simulink model "test_cs"  (Simulink 8.9)
settings: Solver=ode5  StartTime=0.0  StopTime=290  FixedStep=1/20  RelTol=1e-3
model workspace (MAT data in the model file):
  mbox_table.blocks{1}.src = 'built-in/Subsystem'
  mbox_table.blocks{1}.dest = 'test_cs/Audi_A8_1'
  mbox_table.blocks{1}.mode = 0
  mbox_table.blocks{2}.src = 'simulink/Sinks/Out1'
  mbox_table.blocks{2}.dest = 'test_cs/Audi_A8_1/STATE_Audi_A8_1'
  mbox_table.blocks{2}.mode = 0
  mbox_table.blocks{3}.src = 'PreScanSimulinkLibrary/State'
  mbox_table.blocks{3}.dest = 'test_cs/STATE_Audi_A8_1'
  mbox_table.blocks{3}.mode = 0
  mbox_table.blocks{4}.src = 'PreScanSimulinkLibrary/PathFollower'
  mbox_table.blocks{4}.dest = 'test_cs/Audi_A8_1/PathFollower_1'
  mbox_table.blocks{4}.mode = 0
  mbox_table.blocks{5}.src = 'simulink/Sources/Constant'
  mbox_table.blocks{5}.dest = 'test_cs/Audi_A8_1/pos'
  mbox_table.blocks{5}.mode = 0
  mbox_table.blocks{6}.src = 'PreScanSimulinkLibrary/Trajectories'
  mbox_table.blocks{6}.dest = 'test_cs/Audi_A8_1/Trajectories'
  mbox_table.blocks{6}.mode = 0
  mbox_table.blocks{7}.src = 'simulink/Sources/Constant'
  mbox_table.blocks{7}.dest = 'test_cs/Audi_A8_1/Trajectories/Trajectory_1_Offset'
  mbox_table.blocks{7}.mode = 0
  mbox_table.blocks{8}.src = 'PreScanSimulinkLibrary/Trajectory'
  mbox_table.blocks{8}.dest = 'test_cs/Audi_A8_1/Trajectories/Trajectory_1'
  mbox_table.blocks{8}.mode = 0
  mbox_table.blocks{9}.src = 'PreScanSimulinkLibrary/Traj2State'
  mbox_table.blocks{9}.dest = 'test_cs/Audi_A8_1/Trajectories/Traj2State1'
  mbox_table.blocks{9}.mode = 0
  mbox_table.blocks{10}.src = 'simulink/Sinks/Out1'
  mbox_table.blocks{10}.dest = 'test_cs/Audi_A8_1/Trajectories/State'
  mbox_table.blocks{10}.mode = 0
  mbox_table.blocks{11}.src = 'PreScanSimulinkLibrary/SELF'
  mbox_table.blocks{11}.dest = 'test_cs/SELF_Audi_A8_1'
  mbox_table.blocks{11}.mode = 0
  mbox_table.blocks{12}.src = 'simulink/Sources/In1'
  mbox_table.blocks{12}.dest = 'test_cs/Audi_A8_1/SELF_Audi_A8_1'
  mbox_table.blocks{12}.mode = 0
  mbox_table.blocks{13}.src = 'PreScanSimulinkLibrary/DemuxSELF'
  mbox_table.blocks{13}.dest = 'test_cs/Audi_A8_1/SELF_Demux'
  mbox_table.blocks{13}.mode = 0
  mbox_table.blocks{14}.src = 'PreScanSimulinkLibrary/LaneMarkerSensor'
  mbox_table.blocks{14}.dest = 'test_cs/LaneMarkerSensor_1'
  mbox_table.blocks{14}.mode = 0
  mbox_table.blocks{15}.src = 'simulink/Sources/In1'
  mbox_table.blocks{15}.dest = 'test_cs/Audi_A8_1/LaneMarkerSensor_1'
  mbox_table.blocks{15}.mode = 0
  mbox_table.blocks{16}.src = 'PreScanSimulinkLibrary/LaneMarkerSensor_Data'
  mbox_table.blocks{16}.dest = 'test_cs/Audi_A8_1/LaneMarkerSensor_1_Data'
  mbox_table.blocks{16}.mode = 0
  mbox_table.blocks{17}.src = 'PreScanSimulinkLibrary/CameraSensor_Color_Display'
  mbox_table.blocks{17}.dest = 'test_cs/Audi_A8_1/LaneMarkerSensor_1_Display'
  mbox_table.blocks{17}.mode = 0
  mbox_table.blocks{18}.src = 'PreScanSimulinkLibrary/Simple_Vehicle_Dynamics'
  mbox_table.blocks{18}.dest = 'test_cs/Audi_A8_1/Dynamics_Simple'
  mbox_table.blocks{18}.mode = 0
  mbox_table.blocks{19}.src = 'SimCoreLibrary/SimCoreConfiguration'
  mbox_table.blocks{19}.dest = 'test_cs/SimCoreConfiguration'
  mbox_table.blocks{19}.mode = 0
  mbox_table.blocks{20}.src = 'SimCoreLibrary/Actuators'
  mbox_table.blocks{20}.dest = 'test_cs/Actuators'
  mbox_table.blocks{20}.mode = 0
  mbox_table.blocks{21}.src = 'SimCoreLibrary/SetActuators'
  mbox_table.blocks{21}.dest = 'test_cs/SetActuators'
  mbox_table.blocks{21}.mode = 0
  mbox_table.blocks{22}.src = 'SimCoreLibrary/GetSensors'
  mbox_table.blocks{22}.dest = 'test_cs/GetSensors'
  mbox_table.blocks{22}.mode = 0
  mbox_table.blocks{23}.src = 'SimCoreLibrary/SimCoreInfo'
  mbox_table.blocks{23}.dest = 'test_cs/SimCoreInfo'
  mbox_table.blocks{23}.mode = 0
  mbox_table.blocks{24}.src = 'PreScanSimulinkLibrary/Regenerate'
  mbox_table.blocks{24}.dest = 'test_cs/Regenerate'
  mbox_table.blocks{24}.mode = 0
  mbox_table.blocks{25}.src = 'PreScanSimulinkLibrary/Record for Replay  '
  mbox_table.blocks{25}.dest = 'test_cs/Record for Replay  '
  mbox_table.blocks{25}.mode = 0
  mbox_table.blocks{26}.src = 'PreScanSimulinkLibrary/Open Useful Blocks'
  mbox_table.blocks{26}.dest = 'test_cs/Open Useful Blocks'
  mbox_table.blocks{26}.mode = 0
  mbox_table.blocks{27}.src = 'PreScanSimulinkLibrary/PreScan Options   '
  mbox_table.blocks{27}.dest = 'test_cs/PreScan Options   '
  mbox_table.blocks{27}.mode = 0
  mbox_table.blocks{28}.src = 'built-in/Note'
  mbox_table.blocks{28}.dest = 'test_cs/Version:                  '
  mbox_table.blocks{28}.mode = 0
  mbox_table.blocks{29}.src = 'built-in/Note'
  mbox_table.blocks{29}.dest = 'test_cs/7.0.0'
  mbox_table.blocks{29}.mode = 0
  mbox_table.blocks{30}.src = 'built-in/Note'
  mbox_table.blocks{30}.dest = 'test_cs/Author(s):                '
  mbox_table.blocks{30}.mode = 0
  mbox_table.blocks{31}.src = 'built-in/Note'
  mbox_table.blocks{31}.dest = 'test_cs/N.A.'
  mbox_table.blocks{31}.mode = 0
  mbox_table.blocks{32}.src = 'built-in/Note'
  mbox_table.blocks{32}.dest = 'test_cs/Descriptive text:      '
  mbox_table.blocks{32}.mode = 0
  mbox_table.blocks{33}.src = 'built-in/Note'
  mbox_table.blocks{33}.dest = 'test_cs/N.A.'
  mbox_table.blocks{33}.mode = 0
  mbox_table.blocks{34}.src = 'built-in/Note'
  mbox_table.blocks{34}.dest = 'test_cs/ID
    | 
    | 1'
  mbox_table.blocks{34}.mode = 0
  mbox_table.blocks{35}.src = 'built-in/Note'
  mbox_table.blocks{35}.dest = 'test_cs/OBU-Beacon ID
    | 
    | '
  mbox_table.blocks{35}.mode = 0
  mbox_table.blocks{36}.src = 'built-in/Note'
  mbox_table.blocks{36}.dest = 'test_cs/TypeID
    | 
    | 1'
  mbox_table.blocks{36}.mode = 0
  mbox_table.blocks{37}.src = 'built-in/Note'
  mbox_table.blocks{37}.dest = 'test_cs/TypeTag
    | 
    | Car'
  mbox_table.blocks{37}.mode = 0
  mbox_table.blocks{38}.src = 'built-in/Note'
  mbox_table.blocks{38}.dest = 'test_cs/SD
    | 
    | Y'
  mbox_table.blocks{38}.mode = 0
  mbox_table.blocks{39}.src = 'built-in/Note'
  mbox_table.blocks{39}.dest = 'test_cs/CD
    | 
    | N'
  mbox_table.blocks{39}.mode = 0
  mbox_table.blocks{40}.src = 'built-in/Note'
  mbox_table.blocks{40}.dest = 'test_cs/Name
    | 
    | Audi_A8_1'
  mbox_table.blocks{40}.mode = 0
  mbox_table.blocks{41}.src = 'built-in/Note'
  mbox_table.blocks{41}.dest = 'test_cs/Num ID       OBU-Beacon ID     Type ID      Type Tag             SD        CD             Name                          '
  mbox_table.blocks{41}.mode = 0
  mbox_table.blocks{42}.src = 'built-in/Ground'
  mbox_table.blocks{42}.dest = 'test_cs/Audi_A8_1/Ground_1'
  mbox_table.blocks{42}.mode = 1
  mbox_table.blocks{43}.src = 'built-in/Ground'
  mbox_table.blocks{43}.dest = 'test_cs/Audi_A8_1/Ground_2'
  mbox_table.blocks{43}.mode = 1
  mbox_table.blocks{44}.src = 'built-in/Terminator'
  mbox_table.blocks{44}.dest = 'test_cs/Audi_A8_1/Terminator_1'
  mbox_table.blocks{44}.mode = 1
  mbox_table.blocks{45}.src = 'built-in/Terminator'
  mbox_table.blocks{45}.dest = 'test_cs/Audi_A8_1/Terminator_2'
  mbox_table.blocks{45}.mode = 1
  mbox_table.blocks{46}.src = 'built-in/Ground'
  mbox_table.blocks{46}.dest = 'test_cs/Audi_A8_1/Ground_3'
  mbox_table.blocks{46}.mode = 1
  mbox_table.blocks{47}.src = 'built-in/Terminator'
  mbox_table.blocks{47}.dest = 'test_cs/Audi_A8_1/Terminator_3'
  mbox_table.blocks{47}.mode = 1
  mbox_table.blocks{48}.src = 'built-in/Ground'
  mbox_table.blocks{48}.dest = 'test_cs/Audi_A8_1/Ground_4'
  mbox_table.blocks{48}.mode = 1
  mbox_table.blocks{49}.src = 'built-in/Ground'
  mbox_table.blocks{49}.dest = 'test_cs/Audi_A8_1/Ground_5'
  mbox_table.blocks{49}.mode = 1
  mbox_table.blocks{50}.src = 'built-in/Terminator'
  mbox_table.blocks{50}.dest = 'test_cs/Audi_A8_1/Terminator_4'
  mbox_table.blocks{50}.mode = 1
  mbox_table.blocks{51}.src = 'built-in/Terminator'
  mbox_table.blocks{51}.dest = 'test_cs/Audi_A8_1/Terminator_5'
  mbox_table.blocks{51}.mode = 1
  mbox_table.blocks{52}.src = 'built-in/Terminator'
  mbox_table.blocks{52}.dest = 'test_cs/Audi_A8_1/Terminator_6'
  mbox_table.blocks{52}.mode = 1
  mbox_table.blocks{53}.src = 'built-in/Terminator'
  mbox_table.blocks{53}.dest = 'test_cs/Audi_A8_1/Terminator_7'
  mbox_table.blocks{53}.mode = 1
  mbox_table.blocks{54}.src = 'built-in/Terminator'
  mbox_table.blocks{54}.dest = 'test_cs/Audi_A8_1/Terminator_8'
  mbox_table.blocks{54}.mode = 1
  mbox_table.blocks{55}.src = 'built-in/Terminator'
  mbox_table.blocks{55}.dest = 'test_cs/Audi_A8_1/Terminator_9'
  mbox_table.blocks{55}.mode = 1
  mbox_table.blocks{56}.src = 'built-in/Terminator'
  mbox_table.blocks{56}.dest = 'test_cs/Audi_A8_1/Terminator_10'
  mbox_table.blocks{56}.mode = 1
  mbox_table.blocks{57}.src = 'built-in/Terminator'
  mbox_table.blocks{57}.dest = 'test_cs/Audi_A8_1/Terminator_11'
  mbox_table.blocks{57}.mode = 1
  mbox_table.blocks{58}.src = 'built-in/Terminator'
  mbox_table.blocks{58}.dest = 'test_cs/Audi_A8_1/Terminator_12'
  mbox_table.blocks{58}.mode = 1
  mbox_table.blocks{59}.src = 'built-in/Terminator'
  mbox_table.blocks{59}.dest = 'test_cs/Audi_A8_1/Terminator_13'
  mbox_table.blocks{59}.mode = 1
  mbox_table.blocks{60}.src = 'built-in/Terminator'
  mbox_table.blocks{60}.dest = 'test_cs/Audi_A8_1/Terminator_14'
  mbox_table.blocks{60}.mode = 1
  mbox_table.block_index : java.util.Hashtable (value not decoded)
  mbox_table.lines{1}.sys = 'test_cs'
  mbox_table.lines{1}.line_id = 'L1'
  mbox_table.lines{1}.iport = 'STATE_Audi_A8_1/1'
  mbox_table.lines{1}.oport = 'Audi_A8_1/1'
  mbox_table.lines{1}.mode = 0
  mbox_table.lines{2}.sys = 'test_cs/Audi_A8_1'
  mbox_table.lines{2}.line_id = 'L2'
  mbox_table.lines{2}.iport = 'PathFollower_1/1'
  mbox_table.lines{2}.oport = 'pos/1'
  mbox_table.lines{2}.mode = 0
  mbox_table.lines{3}.sys = 'test_cs/Audi_A8_1/Trajectories'
  mbox_table.lines{3}.line_id = 'L3'
  mbox_table.lines{3}.iport = 'Traj2State1/1'
  mbox_table.lines{3}.oport = 'Trajectory_1/1'
  mbox_table.lines{3}.mode = 0
  mbox_table.lines{4}.sys = 'test_cs/Audi_A8_1/Trajectories'
  mbox_table.lines{4}.line_id = 'L4'
  mbox_table.lines{4}.iport = 'Traj2State1/2'
  mbox_table.lines{4}.oport = 'Trajectory_1_Offset/1'
  mbox_table.lines{4}.mode = 0
  mbox_table.lines{5}.sys = 'test_cs/Audi_A8_1/Trajectories'
  mbox_table.lines{5}.line_id = 'L5'
  mbox_table.lines{5}.iport = 'State/1'
  mbox_table.lines{5}.oport = 'Traj2State1/1'
  mbox_table.lines{5}.mode = 0
  mbox_table.lines{6}.sys = 'test_cs'
  mbox_table.lines{6}.line_id = 'L6'
  mbox_table.lines{6}.iport = 'Audi_A8_1/1'
  mbox_table.lines{6}.oport = 'SELF_Audi_A8_1/1'
  mbox_table.lines{6}.mode = 0
  mbox_table.lines{7}.sys = 'test_cs/Audi_A8_1'
  mbox_table.lines{7}.line_id = 'L7'
  mbox_table.lines{7}.iport = 'SELF_Demux/1'
  mbox_table.lines{7}.oport = 'SELF_Audi_A8_1/1'
  mbox_table.lines{7}.mode = 0
  mbox_table.lines{8}.sys = 'test_cs/Audi_A8_1'
  mbox_table.lines{8}.line_id = 'L8'
  mbox_table.lines{8}.iport = 'LaneMarkerSensor_1_Display/1'
  mbox_table.lines{8}.oport = 'LaneMarkerSensor_1_Data/2'
  mbox_table.lines{8}.mode = 0
  mbox_table.lines{9}.sys = 'test_cs/Audi_A8_1'
  mbox_table.lines{9}.line_id = 'L9'
  mbox_table.lines{9}.iport = 'LaneMarkerSensor_1_Display/2'
  mbox_table.lines{9}.oport = 'LaneMarkerSensor_1_Data/3'
  mbox_table.lines{9}.mode = 0
  mbox_table.lines{10}.sys = 'test_cs/Audi_A8_1'
  mbox_table.lines{10}.line_id = 'L10'
  mbox_table.lines{10}.iport = 'LaneMarkerSensor_1_Display/3'
  mbox_table.lines{10}.oport = 'LaneMarkerSensor_1_Data/4'
  mbox_table.lines{10}.mode = 0
  mbox_table.lines{11}.sys = 'test_cs/Audi_A8_1'
  mbox_table.lines{11}.line_id = 'L11'
  mbox_table.lines{11}.iport = 'LaneMarkerSensor_1_Data/1'
  mbox_table.lines{11}.oport = 'LaneMarkerSensor_1/1'
  mbox_table.lines{11}.mode = 0
  mbox_table.lines{12}.sys = 'test_cs'
  mbox_table.lines{12}.line_id = 'L12'
  mbox_table.lines{12}.iport = 'Audi_A8_1/2'
  mbox_table.lines{12}.oport = 'LaneMarkerSensor_1/1'
  mbox_table.lines{12}.mode = 0
  mbox_table.lines{13}.sys = 'test_cs/Audi_A8_1'
  mbox_table.lines{13}.line_id = 'l9'
  mbox_table.lines{13}.iport = 'Dynamics_Simple/1'
  mbox_table.lines{13}.oport = 'PathFollower_1/1'
  mbox_table.lines{13}.mode = 0
  mbox_table.lines{14}.sys = 'test_cs/Audi_A8_1'
  mbox_table.lines{14}.line_id = 'L14'
  mbox_table.lines{14}.iport = 'Dynamics_Simple/2'
  mbox_table.lines{14}.oport = 'PathFollower_1/2'
  mbox_table.lines{14}.mode = 0
  mbox_table.lines{15}.sys = 'test_cs/Audi_A8_1'
  mbox_table.lines{15}.line_id = 'L15'
  mbox_table.lines{15}.iport = 'Dynamics_Simple/3'
  mbox_table.lines{15}.oport = 'PathFollower_1/3'
  mbox_table.lines{15}.mode = 0
  mbox_table.lines{16}.sys = 'test_cs/Audi_A8_1'
  mbox_table.lines{16}.line_id = 'L16'
  mbox_table.lines{16}.iport = 'Dynamics_Simple/4'
  mbox_table.lines{16}.oport = 'PathFollower_1/4'
  mbox_table.lines{16}.mode = 0
  mbox_table.lines{17}.sys = 'test_cs/Audi_A8_1'
  mbox_table.lines{17}.line_id = 'L17'
  mbox_table.lines{17}.iport = 'Dynamics_Simple/6'
  mbox_table.lines{17}.oport = 'PathFollower_1/5'
  mbox_table.lines{17}.mode = 0
  mbox_table.lines{18}.sys = 'test_cs/Audi_A8_1'
  mbox_table.lines{18}.line_id = 'L18'
  mbox_table.lines{18}.iport = 'STATE_Audi_A8_1/1'
  mbox_table.lines{18}.oport = 'Dynamics_Simple/1'
  mbox_table.lines{18}.mode = 0
  mbox_table.lines{19}.sys = 'test_cs/Audi_A8_1'
  mbox_table.lines{19}.line_id = 'l1'
  mbox_table.lines{19}.iport = 'Dynamics_Simple/5'
  mbox_table.lines{19}.oport = 'Ground_1/1'
  mbox_table.lines{19}.mode = 1
  mbox_table.lines{20}.sys = 'test_cs/Audi_A8_1'
  mbox_table.lines{20}.line_id = 'l2'
  mbox_table.lines{20}.iport = 'Dynamics_Simple/7'
  mbox_table.lines{20}.oport = 'Ground_2/1'
  mbox_table.lines{20}.mode = 1
  mbox_table.lines{21}.sys = 'test_cs/Audi_A8_1'
  mbox_table.lines{21}.line_id = 'l3'
  mbox_table.lines{21}.iport = 'Terminator_1/1'
  mbox_table.lines{21}.oport = 'Dynamics_Simple/2'
  mbox_table.lines{21}.mode = 1
  mbox_table.lines{22}.sys = 'test_cs/Audi_A8_1'
  mbox_table.lines{22}.line_id = 'l4'
  mbox_table.lines{22}.iport = 'Terminator_2/1'
  mbox_table.lines{22}.oport = 'Dynamics_Simple/3'
  mbox_table.lines{22}.mode = 1
  mbox_table.lines{23}.sys = 'test_cs/Audi_A8_1'
  mbox_table.lines{23}.line_id = 'l5'
  mbox_table.lines{23}.iport = 'Gain4/1'
  mbox_table.lines{23}.oport = 'Ground_3/1'
  mbox_table.lines{23}.mode = 1
  mbox_table.lines{24}.sys = 'test_cs/Audi_A8_1'
  mbox_table.lines{24}.line_id = 'l6'
  mbox_table.lines{24}.iport = 'Terminator_3/1'
  mbox_table.lines{24}.oport = 'Gain4/1'
  mbox_table.lines{24}.mode = 1
  mbox_table.lines{25}.sys = 'test_cs/Audi_A8_1'
  mbox_table.lines{25}.line_id = 'l7'
  mbox_table.lines{25}.iport = 'PathFollower_1/2'
  mbox_table.lines{25}.oport = 'Ground_4/1'
  mbox_table.lines{25}.mode = 1
  mbox_table.lines{26}.sys = 'test_cs/Audi_A8_1'
  mbox_table.lines{26}.line_id = 'l8'
  mbox_table.lines{26}.iport = 'PathFollower_1/4'
  mbox_table.lines{26}.oport = 'Ground_5/1'
  mbox_table.lines{26}.mode = 1
  mbox_table.lines{27}.sys = 'test_cs/Audi_A8_1'
  mbox_table.lines{27}.line_id = 'l9'
  mbox_table.lines{27}.iport = 'Terminator_4/1'
  mbox_table.lines{27}.oport = 'PathFollower_1/1'
  mbox_table.lines{27}.mode = 1
  mbox_table.lines{28}.sys = 'test_cs/Audi_A8_1'
  mbox_table.lines{28}.line_id = 'l10'
  mbox_table.lines{28}.iport = 'Terminator_5/1'
  mbox_table.lines{28}.oport = 'PathFollower_1/6'
  mbox_table.lines{28}.mode = 1
  mbox_table.lines{29}.sys = 'test_cs/Audi_A8_1'
  mbox_table.lines{29}.line_id = 'l11'
  mbox_table.lines{29}.iport = 'Terminator_6/1'
  mbox_table.lines{29}.oport = 'PathFollower_1/7'
  mbox_table.lines{29}.mode = 1
  mbox_table.lines{30}.sys = 'test_cs/Audi_A8_1'
  mbox_table.lines{30}.line_id = 'l12'
  mbox_table.lines{30}.iport = 'Terminator_7/1'
  mbox_table.lines{30}.oport = 'SELF_Demux/3'
  mbox_table.lines{30}.mode = 1
  mbox_table.lines{31}.sys = 'test_cs/Audi_A8_1'
  mbox_table.lines{31}.line_id = 'l13'
  mbox_table.lines{31}.iport = 'Terminator_8/1'
  mbox_table.lines{31}.oport = 'SELF_Demux/4'
  mbox_table.lines{31}.mode = 1
  mbox_table.lines{32}.sys = 'test_cs/Audi_A8_1'
  mbox_table.lines{32}.line_id = 'l14'
  mbox_table.lines{32}.iport = 'Terminator_9/1'
  mbox_table.lines{32}.oport = 'SELF_Demux/5'
  mbox_table.lines{32}.mode = 1
  mbox_table.lines{33}.sys = 'test_cs/Audi_A8_1'
  mbox_table.lines{33}.line_id = 'l15'
  mbox_table.lines{33}.iport = 'Terminator_10/1'
  mbox_table.lines{33}.oport = 'SELF_Demux/7'
  mbox_table.lines{33}.mode = 1
  mbox_table.lines{34}.sys = 'test_cs/Audi_A8_1'
  mbox_table.lines{34}.line_id = 'l16'
  mbox_table.lines{34}.iport = 'Terminator_11/1'
  mbox_table.lines{34}.oport = 'SELF_Demux/8'
  mbox_table.lines{34}.mode = 1
  mbox_table.lines{35}.sys = 'test_cs/Audi_A8_1'
  mbox_table.lines{35}.line_id = 'l17'
  mbox_table.lines{35}.iport = 'Terminator_12/1'
  mbox_table.lines{35}.oport = 'SELF_Demux/9'
  mbox_table.lines{35}.mode = 1
  mbox_table.lines{36}.sys = 'test_cs/Audi_A8_1'
  mbox_table.lines{36}.line_id = 'l18'
  mbox_table.lines{36}.iport = 'Terminator_13/1'
  mbox_table.lines{36}.oport = 'SELF_Demux/11'
  mbox_table.lines{36}.mode = 1
  mbox_table.lines{37}.sys = 'test_cs/Audi_A8_1'
  mbox_table.lines{37}.line_id = 'l19'
  mbox_table.lines{37}.iport = 'Terminator_14/1'
  mbox_table.lines{37}.oport = 'Trajectories/1'
  mbox_table.lines{37}.mode = 1
  mbox_table.line_index : java.util.Hashtable (value not decoded)
  mbox_table.next_linenr = 19
  mbox_table.next_termlinenr = 20
  model_closed = 0
  sim_status = 0
PreLoadFcn:
  | check_NUTS_defined;
  | 
  | assignin('base',['model_closed_' bdroot],false);
InitFcn:
  | PreScanExperimentInitFcn(bdroot)
StopFcn:
  | PreScanExperimentStopFcn(bdroot)
values from neighbouring files (symbols this model uses):
  a11 = -2*(cf*Lf^2+cr*Lr^2)/(Iz*Vx)    (= -13.1812002432)    [lkas.m]
  a12 = 2*(cf*Lf-cr*Lr)/Iz    (= -69.3863961559)    [lkas.m]
  a13 = -2*(cf*Lf-cr*Lr)/(Iz*Vx)    (= 3.56925906152)    [lkas.m]
  a16 = 2*cf*Lf/Iz    (= 45.3838814736)    [lkas.m]
  a31 = 2*(-cf*Lf+cr*Lr)/(M*Vx)    (= 7.3463980464)    [lkas.m]
  a32 = 2*(cf+cr)/M    (= 213.298901099)    [lkas.m]
  a33 = -2*(cf+cr)/(M*Vx)    (= -10.9721656944)    [lkas.m]
  a36 = 2*cf/M    (= 79.8384615385)    [lkas.m]
  K = acker(A, B, [-10+10i -10-10i -10 -10])    [lkas.m]
  L = L'    [lkas.m]
undefined symbols (not defined in the file or in its folder): InitImageOutputDir
libraries: simulink x18, PreScanSimulinkLibrary x6, simulink_extras x3
(part 1 of 3)
CloseFcn:
  | evalin('base',['clear model_closed_' bdroot]);
settings Model: Creator=PRESCAN  LastModifiedBy=edward
settings OptimizationCC: ExpressionDepthLimit=2147483647  InitFltsAndDblsToZero=on
settings DebuggingCC: SaveWithParameterizedLinksMsg=none  SignalResolutionControl=TryResolveAllWithWarning  MultiTaskDSMMsg=warning  MultiTaskCondExecSysMsg=none
settings GRTTargetCC: TargetFcnLib=ansi_tfl_tmw.mat

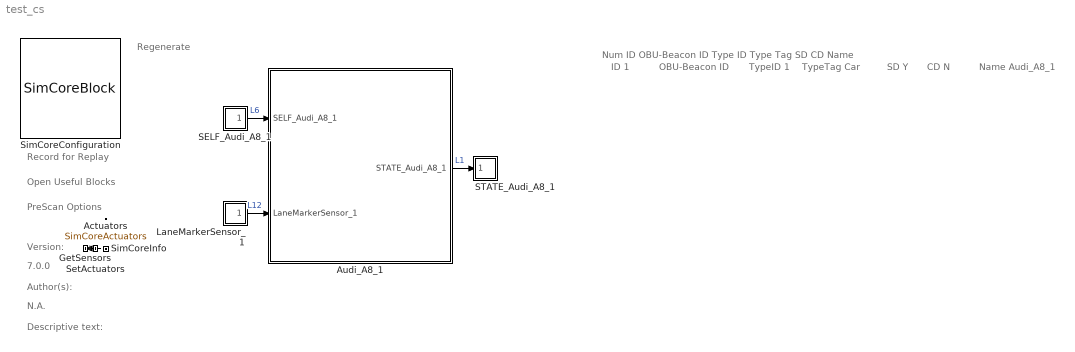
== system test_cs ==
  note: Regenerate
  note: Record for Replay
  note: Open Useful Blocks
  note: PreScan Options
  note: Version:
  note: 7.0.0
  note: Author(s):
  note: N.A.
  note: Descriptive text:
  note: ID
      |
      | 1
  note: OBU-Beacon ID
  note: TypeID
      |
      | 1
  note: TypeTag
      |
      | Car
  note: SD
      |
      | Y
  note: CD
      |
      | N
  note: Name
      |
      | Audi_A8_1
  note: Num ID OBU-Beacon ID Type ID Type Tag SD CD Name
  Actuators : DataStoreMemory  DataStoreName=SimCoreActuators  InitialValue=zeros(15,1)  ShowAdditionalParam=off
  Audi_A8_1 : Subsystem  Tag=WorldObjectSubSystem  InitFcn=UniqueId = '13';
      mask Display: image(imread('Audi_A8.jpg'));color('white');text(0,0,' ID=1\n')
  GetSensors : Subsystem  Tag=GetSensors  mask(PreScan Simulation Core Block){NrOfSensors=8, TimeStep=1/20}
      mask prompts: NrOfSensors "Number of sensor values"; TimeStep "Timestep [s]"
      mask help:
      | Please do not remove this block from the PreScan compilation sheet,
      | as it contains essential configuration parameters for a PreScan simulation.
      settings: DeleteFcn=PreScanBlockDeleteFcn;
  LaneMarkerSensor_1 : Subsystem  Tag=LaneMarkerSensor  mask(PreScan Source Block: Lane Marker Sensor){}
      mask help: The Lane Marker Sensor provides information relating the sensor to the lane markers on the road.
      settings: DeleteFcn=PreScanBlockDeleteFcn;
      mask Help: eval('openHelp(457)')
      mask Display: image(imread('LaneMarkerSensorSL.png'))
  SELF_Audi_A8_1 : Subsystem  Tag=SELF  mask(PreScan Source Block: SELF){PortName=SELF_Audi_A8_1, PortIndex=0, PortWidth=8, TimeStep=1/20}
      mask prompts: PortName "Auto-Assigned: Port Name [-]"; PortIndex "Auto-Assigned: Port Index [-]"; PortWidth "Auto-Assigned: Port Dimensions"; TimeStep "Auto-Assigned: Upload Period [s]"
      mask help:
      | The SELF port shows (state) information of the actor itself. The outputs are position in the experiment's axis system and the GPS coordinates, and the object's absolute velocity and compass heading.
      |
      | For more information, please click Help.
      settings: DeleteFcn=PreScanBlockDeleteFcn;
      mask Help: eval('openHelp(462)')
      mask Display: image(imread('GPS.png'))
  STATE_Audi_A8_1 : Subsystem  Tag=State  mask(PreScan Sink Block: State){x0=-466.9761730372511, y0=-32.058094010780337, z0=0.55, Roll0=0, Pitch0=0, Yaw0=0, TimeStep=1/20}
      mask prompts: x0 "Ini x-position VEHICLE wrt GLOBAL axis system [m]"; y0 "Ini y-position VEHICLE wrt GLOBAL axis system [m]"; z0 "Ini z-position VEHICLE wrt GLOBAL axis system [m]"; Roll0 "Ini roll-angle BODY wrt VEHICLE axis system [deg]"; Pitch0 "Ini pitch-angle BODY wrt VEHICLE axis system [deg]"; Yaw0 "Ini yaw-angle VEHICLE wrt GLOBAL axis system [deg]"; TimeStep "Time Step [s]"
      mask help:
      | The Actor State contains a vector signal of size (9x1), containing the following signals:
      |
      | -  Position                  (x,y,z)                                     [m]
      | -  Velocity                  (vx,vy,vz)                               [m/s]
      | -  Angles                    (Roll, Pitch, Yaw)                   [rad]
      |
      | The Actor state is defined in the global axis system.
      | The state is superponed on the Initial position defined in the GUI.
      |
      | For more information, please click Help.
      settings: DeleteFcn=PreScanBlockDeleteFcn;
      mask Help: eval('openHelp(222)')
      mask Display: image(imread('State.png'))
  SetActuators : Subsystem  Tag=SetActuators  mask(PreScan Simulation Core Block){TimeStep=1/20, NrOfActuators=15}
      mask prompts: TimeStep "Timestep [s]"; NrOfActuators "Number of actuator values"
      mask help:
      | Please do not remove this block from the PreScan compilation sheet,
      | as it contains essential configuration parameters for a PreScan simulation.
      settings: DeleteFcn=PreScanBlockDeleteFcn;
  SimCoreConfiguration : M-S-Function  Tag=SimCoreConfiguration  Description=FE4822352E09E935CCF95F68F07A56B5C1887AE4C351415F02894CADC90007F4  FunctionName=SimCoreBlock  Parameters=ExperimentXML PortsXML SimulationCore HostName CheckStart EnableLog RfR EnableGPUAccel ShowComputationTime  mask(PreScan Simulation Core Configurator){SimulationCore=NUTS, HostName=0, CheckStart=0, prescanversion='7.0.0', EnableLog=off, RfR=0, EnableGPUAccel=off, ShowComputationTime=off}
      mask prompts: SimulationCore "Simulation Core"; HostName "Simulation Host"; CheckStart "Show START Dialog"; prescanversion "PreScan Version"; EnableLog "Create TA Log"; RfR "Record for Replay"; EnableGPUAccel "Enable GPU Acceleration"; ShowComputationTime "Show ComputationTime Scope"
      mask help:
      | Please do not remove this block from the PreScan compilation sheet,
      | as it contains essential configuration parameter for a PreScan simulation.
      mask init:
      | model = bdroot;
      | ExperimentXML = [model(1:end-3) '.pex'];
      | PortsXML = [model '_ports.pcd'];
      settings: DeleteFcn=PreScanBlockDeleteFcn;  ModelCloseFcn=assignin('base',['model_closed_' bdroot],true);
      mask Help: eval('openHelp(812)')
      mask Display: image(imread('prescanlogo.ico'))
  SimCoreInfo : Subsystem  Tag=SimCoreInfo
  wires:
  SetActuators/1(dummy) -> GetSensors/1(dummy)
  Audi_A8_1/1(STATE_Audi_A8_1) -> STATE_Audi_A8_1/1(State)  "L1"
  SELF_Audi_A8_1/1(U) -> Audi_A8_1/1(SELF_Audi_A8_1)  "L6"
  LaneMarkerSensor_1/1(U) -> Audi_A8_1/2(LaneMarkerSensor_1)  "L12"

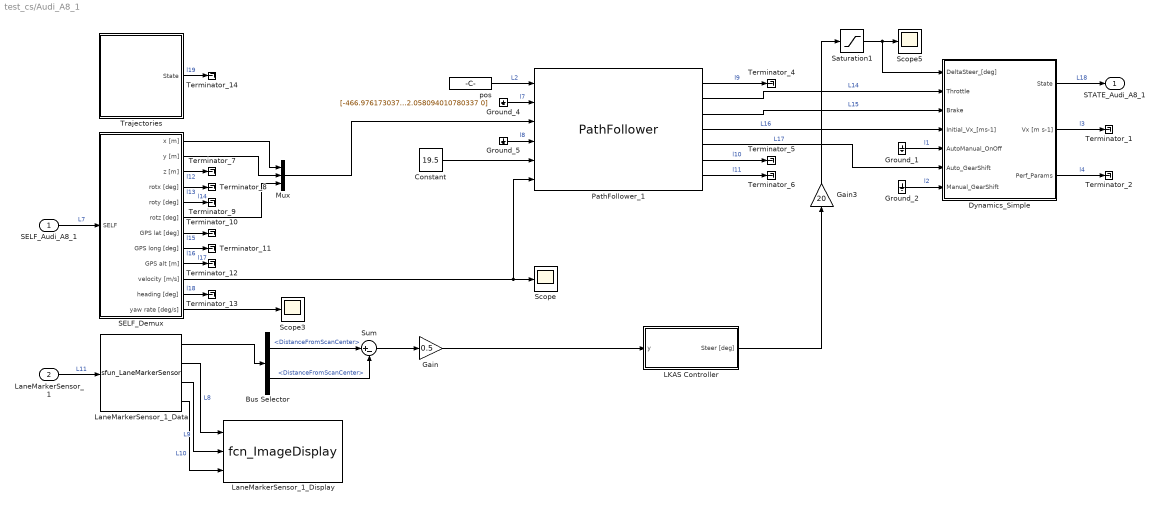
== system test_cs/Audi_A8_1 ==
  SELF_Audi_A8_1 : Inport  Tag=SELFInport
  LaneMarkerSensor_1 : Inport  Tag=LaneMarkerSensorInport  Port=2  SampleTime=1/20
  Bus Selector : BusSelector  OutputSignals=ScanAtDistance1.LeftCurbIntersection.DistanceFromScanCenter,ScanAtDistance1.RightCurbIntersection.DistanceFromScanCenter
  Constant : Constant  Value=19.5
  Dynamics_Simple : Subsystem  Tag=Simple_Vehicle_Dynamics  mask(PreScan Block: Simple Dynamics){TimeStep=1/20, ComputationMode=Continuous_Time}
      mask prompts: TimeStep "Auto assigned: Time Step [s]"; ComputationMode "Computation mode:"
      mask help:
      | The Simple Dynamics Model is selected in the GUI to simulate vehicle dynamics behavior.
      |
      | The Simple Dynamics Model is completely open to the user. The parameters of this model can be set in the Simple Dynamics dialog in the GUI.
      |
      | For more information, please click Help.
      mask init:
      | p = SimpleDyn_pars;
      settings: DeleteFcn=PreScanBlockDeleteFcn;
      mask Help: eval('openHelp(220)')
      mask Display:
      | image(imread('SimpleDyn.png'))
      | port_label('input', 1, '{\delta}_S_t_ _e_e_r [deg]','texmode','on')
      | port_label('input', 2, 'Throttle [%]')
      | port_label('input', 3, 'Brake Pres [bar]')
      | port_label('input', 4, 'V_0 [ms-1]','texmode','on')
      | port_label('input', 5, 'Auto=[0]/Manual=[1]')
      | port_label('input', 6, 'Auto_GearShift')
      | port_label('input', 7, 'Manual_GearShift')
      | port_label('output', 1, 'State')
      | port_label('output', 2, 'Vx [ms-1]')
      | port_label('output', 3, 'Perf Params')
  Gain : Gain  Gain=0.5
  Gain3 : Gain  Gain=20
  Ground_{1..2,4..5} (4 alike) : Ground
  LKAS Controller : Subsystem
  LaneMarkerSensor_1_Data : S-Function  Tag=LaneMarkerSensor_Data  LoadFcn=load('LaneMarkerSensorBusses.mat');  FunctionName=sfun_LaneMarkerSensor  Parameters=[VerticalResolution HorizontalResolution] FrameRate SensorName OutputReferenceImage SharedMemTag SharedMemDataTag  SFunctionDeploymentMode=off  EnableBusSupport=on  mask{HorizontalResolution=320, VerticalResolution=240, FrameRate=20, SensorName=LaneMarkerSensor_1, OutputReferenceImage=on, SharedMemTag=LaneMarkerSensor_1_monoBeam_viewer_RGB, SharedMemDataTag=LaneMarkerSensor_1_monoBeam_viewer_LMS_Data}
      mask prompts: HorizontalResolution "User Specified: Horizontal Resolution [pixels]"; VerticalResolution "User Specified: Vertical Resolution [pixels]"; FrameRate "User Specified: Frame Rate [Hz]"; SensorName "User Specified: Lane Marker Sensor Name"; OutputReferenceImage "User Specified: Output Reference Image"; SharedMemTag "Tag for shared memory for lane marker img"; SharedMemDataTag "Tag for shared memory data"
      mask init:
      | DataPort = 1;
      | if OutputReferenceImage==1
      |     Rport = 2;
      |     Gport = 3;
      |     Bport = 4;
      |     RportName = 'Ref. Image R';
      |     GportName = 'Ref. Image G';
      |     BportName = 'Ref. Image B';
      | else
      |     Rport = 1;
      |     Gport = 1;
      |     Bport = 1;
      |     RportName = '';
      |     GportName = '';
      |     BportName = '';
      | end
      settings: DeleteFcn=PreScanBlockDeleteFcn;
      mask Display:
      | port_label('output',DataPort,'Detection Data')
      | port_label('output',Rport,RportName)
      | port_label('output',Gport,GportName)
      | port_label('output',Bport,BportName)
  LaneMarkerSensor_1_Display : M-S-Function  Tag=CameraSensor_Color_Display  InitFcn=InitImageOutputDir(gcb);  FunctionName=fcn_ImageDisplay  Parameters=SensorName EnableDisplay EnablePosition DisplayPosition FigureHandle SaveResults BitmapFormat TempOutputDir CameraType  mask(PreScan Color Display Block){SensorName=LaneMarkerSensor_1, EnableDisplay=on, EnablePosition=off, DisplayPosition=[10 10 320 240], FigureHandle=100, SaveResults=off, Format=PNG, TempOutputDir=0, CameraType=Mono}
      mask prompts: SensorName "User Specified: Title of Display"; EnableDisplay "Active"; EnablePosition "Set Display window position"; DisplayPosition "Display window position [xpos ypos width height]"; FigureHandle "Unique Handle"; SaveResults "Save results"; TempOutputDir "OutputDir"; CameraType "Camera Type"
      mask help: This block displays the RGB output of a PreScan camera sensor.
      mask init:
      | if EnableDisplay
      |     EnableString='';
      |     EnableColor='gray';
      | else
      |     EnableString='INACTIVE';
      |     EnableColor='red';
      | end
      | switch Format
      |     case 1
      |         BitmapFormat = 'png';
      |     case 2
      |         BitmapFormat = 'bmp';
      |     case 3
      |         BitmapFormat = 'jpg';
      | end 
      | if CameraType==1
      |     CameraTypeName='MONO';
      |     PortNumber=0;
      | else
      |     CameraTypeName='STEREO';
      |     PortNumber=3;
      | end
      settings: DeleteFcn=PreScanBlockDeleteFcn;  ModelCloseFcn=fcn_ImageDisplay_ModelCloseFcn
      mask Help: eval('openHelp(457)')
      mask Callback EnablePosition:
      | MV=get_param(gcb,'MaskVisibilities');
      | if strcmp(get_param(gcb,'EnablePosition'),'on')
      |     MV{4}='on';
      | else
      |     MV{4}='off';
      | end
      | set_param(gcb,'MaskVisibilities',MV);
      mask TypeOptions Format: PNG | BMP | JPG
      mask TypeOptions CameraType: Mono | Stereo
      mask Display:
      | color(EnableColor);
      | fprintf('%s\n DISPLAY:\n Color \n %s',EnableString,SensorName)
      | port_label('input',1,'R')
      | port_label('input',2,'G')
      | port_label('input',3,'B')
      | port_label('input',PortNumber+1,'R')
      | port_label('input',PortNumber+2,'G')
      | port_label('input',PortNumber+3,'B')
  Mux : Mux  Inputs=3
  PathFollower_1 : PreScanSimulinkLibrary/PathFollower  Tag=pathFollower  FileName='Trajectory_1.mat'  TunableSteeringGain=1  XShifting_wrt_COG=0
  SELF_Demux : Subsystem  Tag=DemuxSELF  mask(PreScan Demux Block:){}
      settings: DeleteFcn=PreScanBlockDeleteFcn;
      mask Display:
      | port_label('output',1,'x [m]')
      | port_label('output',2,'y [m]')
      | port_label('output',3,'z [m]','texmode','on')
      | port_label('output',4,'Rotx [deg]','texmode','on')
      | port_label('output',5,'Roty [deg]','texmode','on')
      | port_label('output',6,'Rotz [deg]','texmode','on')
      | port_label('output',7,'GPS lat [deg]','texmode','on')
      | port_label('output',8,'GPS long [deg]','texmode','on')
      | port_label('output',9,'GPS alt [m]','texmode','on')
      | port_label('output',10,'Velocity [m/s]')
      | port_label('output',11,'Heading [deg]')
      | port_label('output',12,'Yaw rate [deg/s]')
  Saturation1 : Saturate  UpperLimit=400  LowerLimit=-400
  Scope : Scope
  Scope3 : Scope
  Scope5 : Scope
  Sum : Sum  Inputs=|+-
  Terminator_{1..2,4..14} (13 alike) : Terminator
  Trajectories : Subsystem  Tag=Trajectories  mask(PreScan Source Block: Trajectories){}
      mask help:
      | The Trajectory block contains the trajectories defined in the PreScan Experiment Editor. The output of the trajectory block is the (vehicle) State.
      |
      | For more information, please click Help.
      settings: DeleteFcn=PreScanBlockDeleteFcn;
      mask Help: eval('openHelp(312)')
      mask Display: image(imread('Trajectory.png'));
  pos : Constant  Tag=pos  Value=[-466.9761730372511 -32.058094010780337 0]
  STATE_Audi_A8_1 : Outport  Tag=StateOutport
  wires:
  LaneMarkerSensor_1_Data/1 -> Bus Selector/1
  Mux/1 -> PathFollower_1/3
  SELF_Demux/1(x [m]) -> Mux/1
  SELF_Demux/2(y [m]) -> Mux/2
  SELF_Demux/6(rotz [deg]) -> Mux/3
  SELF_Demux/10(velocity [m/s]) -> PathFollower_1/6, Scope/1
  Bus Selector/1 -> Sum/1  "<DistanceFromScanCenter>"
  Bus Selector/2 -> Sum/2  "<DistanceFromScanCenter>"
  Sum/1 -> Gain/1
  Constant/1 -> PathFollower_1/5
  Gain3/1 -> Saturation1/1
  Saturation1/1 -> Scope5/1, Dynamics_Simple/1(DeltaSteer_[deg])
  SELF_Demux/12(yaw rate [deg/s]) -> Scope3/1
  pos/1 -> PathFollower_1/1  "L2"
  SELF_Audi_A8_1/1 -> SELF_Demux/1(SELF)  "L7"
  LaneMarkerSensor_1_Data/2 -> LaneMarkerSensor_1_Display/1  "L8"
  LaneMarkerSensor_1_Data/3 -> LaneMarkerSensor_1_Display/2  "L9"
  LaneMarkerSensor_1_Data/4 -> LaneMarkerSensor_1_Display/3  "L10"
  LaneMarkerSensor_1/1 -> LaneMarkerSensor_1_Data/1  "L11"
  PathFollower_1/2 -> Dynamics_Simple/2(Throttle)  "L14"
  PathFollower_1/3 -> Dynamics_Simple/3(Brake)  "L15"
  PathFollower_1/4 -> Dynamics_Simple/4(Initial_Vx_[ms-1])  "L16"
  PathFollower_1/5 -> Dynamics_Simple/6(Auto_GearShift)  "L17"
  Dynamics_Simple/1(State) -> STATE_Audi_A8_1/1  "L18"
  Ground_1/1 -> Dynamics_Simple/5(AutoManual_OnOff)  "l1"
  Ground_2/1 -> Dynamics_Simple/7(Manual_GearShift)  "l2"
  Dynamics_Simple/2(Vx [m s-1]) -> Terminator_1/1  "l3"
  Dynamics_Simple/3(Perf_Params) -> Terminator_2/1  "l4"
  Ground_4/1 -> PathFollower_1/2  "l7"
  Ground_5/1 -> PathFollower_1/4  "l8"
  PathFollower_1/1 -> Terminator_4/1  "l9"
  PathFollower_1/6 -> Terminator_5/1  "l10"
  PathFollower_1/7 -> Terminator_6/1  "l11"
  SELF_Demux/3(z [m]) -> Terminator_7/1  "l12"
  SELF_Demux/4(rotx [deg]) -> Terminator_8/1  "l13"
  SELF_Demux/5(roty [deg]) -> Terminator_9/1  "l14"
  SELF_Demux/7(GPS lat [deg]) -> Terminator_10/1  "l15"
  SELF_Demux/8(GPS long [deg]) -> Terminator_11/1  "l16"
  SELF_Demux/9(GPS alt [m]) -> Terminator_12/1  "l17"
  SELF_Demux/11(heading [deg]) -> Terminator_13/1  "l18"
  Trajectories/1(State) -> Terminator_14/1  "l19"
  Gain/1 -> LKAS Controller/1(y)
  LKAS Controller/1(Steer [deg]) -> Gain3/1

== system test_cs/GetSensors ==
  dummy : Inport
  GetSensors : M-S-Function  FunctionName=GetSensorsBlock  Parameters=TimeStep NrOfSensors
  tag scope: SimCoreSensors=global
  wires:
  GetSensors/1 -> [SimCoreSensors]
  dummy/1 -> GetSensors/1

== system test_cs/LaneMarkerSensor_1 ==
  Demux : Demux  Outputs=[1 -1]
  Terminator : Terminator
  U : Outport
  wires:
  Demux/2 -> Terminator/1
  Demux/1 -> U/1
  [SimCoreSensors] -> Demux/1

== system test_cs/SELF_Audi_A8_1 ==
  Selector : Selector  IndexMode=Zero-based  IndexOptions=Starting index (dialog)  Indices=PortIndex  OutputSizes=PortWidth(1)
  U : Outport
  wires:
  Selector/1 -> U/1
  [SimCoreSensors] -> Selector/1

== system test_cs/STATE_Audi_A8_1 ==
  State : Inport  SampleTime=TimeStep
  Acceleration : Subsystem  mask(ToSensorWorld){PortName=Acceleration_Audi_A8_1, PortIndex=6, PortWidth=3, TimeStep=1/20}
      mask prompts: PortName "Port Name [-]"; PortIndex "Index [-]"; PortWidth "Port Dimensions [-]"; TimeStep "Upload Period [s]"
      mask help: Sends signal(s) from Simulink to the Sensor World
      mask Help:
      | Sends signal(s) from Simulink to the Sensor World.
      | 
      | - Port Name [-]: specifies the name of the output terminal of the Simulink block.
      | - Index [-]: specifies the start position in the output vector sent to the Sensor World
      | - Port dimensions [-]: specifies the width (number of scalars) of the output port
      | - Upload period [s]: specifies the upload period (in seconds) of the port.
      mask Display: port_label('input', 1, PortName)
  Demux : Demux  Outputs=5
  Position : Subsystem  mask(ToSensorWorld){PortName=Position_Audi_A8_1, PortIndex=0, PortWidth=3, TimeStep=1/20}
      mask prompts: PortName "Port Name [-]"; PortIndex "Index [-]"; PortWidth "Port Dimensions [-]"; TimeStep "Upload Period [s]"
      mask help: Sends signal(s) from Simulink to the Sensor World
      mask Help:
      | Sends signal(s) from Simulink to the Sensor World.
      | 
      | - Port Name [-]: specifies the name of the output terminal of the Simulink block.
      | - Index [-]: specifies the start position in the output vector sent to the Sensor World
      | - Port dimensions [-]: specifies the width (number of scalars) of the output port
      | - Upload period [s]: specifies the upload period (in seconds) of the port.
      mask Display: port_label('input', 1, PortName)
  RPY : Subsystem  mask(ToSensorWorld){PortName=RPY_Audi_A8_1, PortIndex=9, PortWidth=3, TimeStep=1/20}
      mask prompts: PortName "Port Name [-]"; PortIndex "Index [-]"; PortWidth "Port Dimensions [-]"; TimeStep "Upload Period [s]"
      mask help: Sends signal(s) from Simulink to the Sensor World
      mask Help:
      | Sends signal(s) from Simulink to the Sensor World.
      | 
      | - Port Name [-]: specifies the name of the output terminal of the Simulink block.
      | - Index [-]: specifies the start position in the output vector sent to the Sensor World
      | - Port dimensions [-]: specifies the width (number of scalars) of the output port
      | - Upload period [s]: specifies the upload period (in seconds) of the port.
      mask Display: port_label('input', 1, PortName)
  Velocity : Subsystem  mask(ToSensorWorld){PortName=Velocity_Audi_A8_1, PortIndex=3, PortWidth=3, TimeStep=1/20}
      mask prompts: PortName "Port Name [-]"; PortIndex "Index [-]"; PortWidth "Port Dimensions [-]"; TimeStep "Upload Period [s]"
      mask help: Sends signal(s) from Simulink to the Sensor World
      mask Help:
      | Sends signal(s) from Simulink to the Sensor World.
      | 
      | - Port Name [-]: specifies the name of the output terminal of the Simulink block.
      | - Index [-]: specifies the start position in the output vector sent to the Sensor World
      | - Port dimensions [-]: specifies the width (number of scalars) of the output port
      | - Upload period [s]: specifies the upload period (in seconds) of the port.
      mask Display: port_label('input', 1, PortName)
  iniBODYAngles wrtVEH [rad] : Constant  Value=[Roll0 Pitch0 0]  SampleTime=TimeStep
  iniVEHAngles wrtGLOB [rad] : Constant  Value=[0 0 Yaw0]  SampleTime=TimeStep
  iniVEHposition wrtGLOB [m] : Constant  Value=[x0 y0 z0]  SampleTime=TimeStep
  state2FullState : PreScanSimulinkLibrary/state2FullState  SystemSampleTime=-1
  velRPY : Subsystem  mask(ToSensorWorld){PortName=velRPY_Audi_A8_1, PortIndex=12, PortWidth=3, TimeStep=1/20}
      mask prompts: PortName "Port Name [-]"; PortIndex "Index [-]"; PortWidth "Port Dimensions [-]"; TimeStep "Upload Period [s]"
      mask help: Sends signal(s) from Simulink to the Sensor World
      mask Help:
      | Sends signal(s) from Simulink to the Sensor World.
      | 
      | - Port Name [-]: specifies the name of the output terminal of the Simulink block.
      | - Index [-]: specifies the start position in the output vector sent to the Sensor World
      | - Port dimensions [-]: specifies the width (number of scalars) of the output port
      | - Upload period [s]: specifies the upload period (in seconds) of the port.
      mask Display: port_label('input', 1, PortName)
  wires:
  Demux/5 -> velRPY/1(Y)
  Demux/4 -> RPY/1(Y)
  Demux/3 -> Acceleration/1(Y)
  Demux/2 -> Velocity/1(Y)
  Demux/1 -> Position/1(Y)
  State/1 -> state2FullState/1
  state2FullState/1 -> Demux/1
  iniVEHposition wrtGLOB [m]/1 -> state2FullState/2
  iniBODYAngles wrtVEH [rad]/1 -> state2FullState/3
  iniVEHAngles wrtGLOB [rad]/1 -> state2FullState/4

== system test_cs/SetActuators ==
  Bus Creator : BusCreator  Inputs=1
  Data Store Read : DataStoreRead  DataStoreName=SimCoreActuators  SampleTime=TimeStep
  SendActuators : M-S-Function  FunctionName=SendActuatorsBlock  Parameters=TimeStep NrOfActuators
  dummy : Outport
  tag scope: SimCoreInfo=global
  wires:
  Bus Creator/1 -> [SimCoreInfo]  "SimCore"
  SendActuators/2 -> Bus Creator/1  "ComputationTime[s]"
  SendActuators/1 -> dummy/1
  Data Store Read/1 -> SendActuators/1

== system test_cs/SimCoreInfo ==
  Bus Selector : BusSelector  OutputSignals=ComputationTime[s]
  Time : Scope
  wires:
  Bus Selector/1 -> Time/1  "<ComputationTime[s]>"
  [SimCoreInfo] -> Bus Selector/1

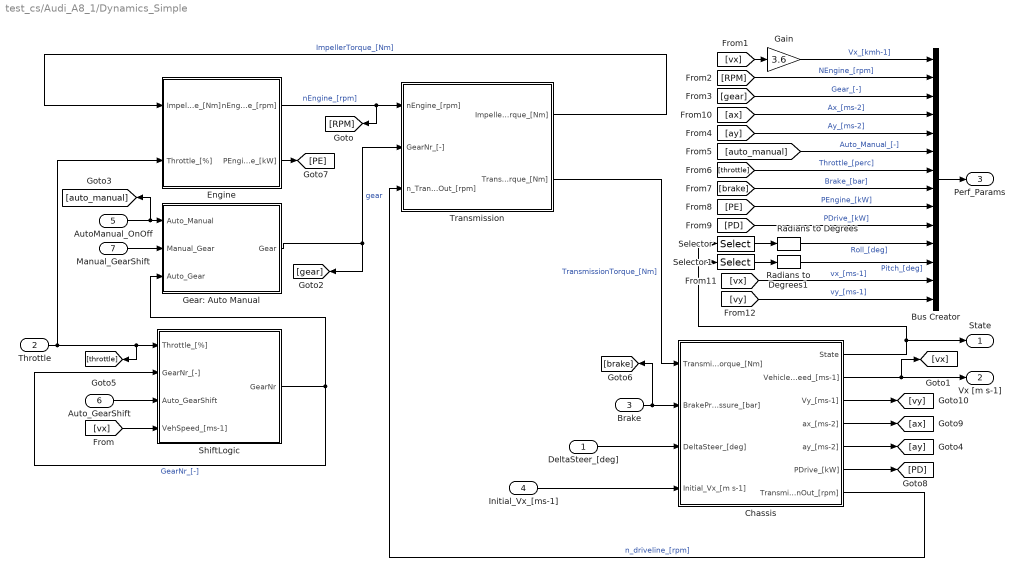
== system test_cs/Audi_A8_1/Dynamics_Simple ==
  DeltaSteer_[deg] : Inport
  Throttle : Inport  Port=2
  Brake : Inport  Port=3
  Initial_Vx_[ms-1] : Inport  Port=4
  AutoManual_OnOff : Inport  Port=5
  Auto_GearShift : Inport  Port=6
  Manual_GearShift : Inport  Port=7
  Bus Creator : BusCreator  Inputs=14
  Chassis : Subsystem
      mask Display: image(imread('Chassis.png'));
  Engine : Subsystem
      mask Display: image(imread('Engine.png'));
  Gain : Gain  Gain=3.6
  Gear: Auto Manual : Subsystem
  Radians to Degrees : simulink_extras/Transformations/Radians to Degrees
  Radians to Degrees1 : simulink_extras/Transformations/Radians to Degrees
  Selector : Selector  InputPortWidth=9  IndexOptions=Index vector (dialog)  Indices=7  OutputSizes=1
  Selector1 : Selector  InputPortWidth=9  IndexOptions=Index vector (dialog)  Indices=8  OutputSizes=1
  ShiftLogic : Subsystem
      mask Display: image(imread('Gearshift.png'));
  Transmission : Subsystem
      mask Display: image(imread('Transmission.png'));
  State : Outport
  Vx [m s-1] : Outport  Port=2
  Perf_Params : Outport  Port=3
  wires:
  [vy] -> Bus Creator/14  "vy_[ms-1]"
  [vx] -> Bus Creator/13  "vx_[ms-1]"
  Chassis/7(TransmissionOut_[rpm]) -> Transmission/3(n_TransmissionOut_[rpm])  "n_driveline_[rpm]"
  Chassis/6(PDrive_[kW]) -> [PD]
  Chassis/5(ay_[ms-2]) -> [ay]
  Chassis/4(ax_[ms-2]) -> [ax]
  Chassis/3(Vy_[ms-1]) -> [vy]
  [vx] -> ShiftLogic/4(VehSpeed_[ms-1])
  Gear: Auto Manual/1(Gear) -> Transmission/2(GearNr_[-]), [gear]  "gear"
  Manual_GearShift/1 -> Gear: Auto Manual/2(Manual_Gear)
  AutoManual_OnOff/1 -> Gear: Auto Manual/1(Auto_Manual), [auto_manual]
  Chassis/2(VehicleSpeed_[ms-1]) -> [vx], Vx [m s-1]/1
  Auto_GearShift/1 -> ShiftLogic/3(Auto_GearShift)
  Throttle/1 -> Engine/2(Throttle_[%]), ShiftLogic/1(Throttle_[%]), [throttle]
  Initial_Vx_[ms-1]/1 -> Chassis/4(Initial_Vx_[m s-1])
  DeltaSteer_[deg]/1 -> Chassis/3(DeltaSteer_[deg])
  Chassis/1(State) -> State/1, Selector/1, Selector1/1
  Brake/1 -> [brake], Chassis/2(BrakePressure_[bar])
  Engine/1(nEngine_[rpm]) -> [RPM], Transmission/1(nEngine_[rpm])  "nEngine_[rpm]"
  ShiftLogic/1(GearNr) -> Gear: Auto Manual/3(Auto_Gear), ShiftLogic/2(GearNr_[-])  "GearNr_[-]"
  Transmission/2(TransmissionTorque_[Nm]) -> Chassis/1(TransmissionTorque_[Nm])  "TransmissionTorque_[Nm]"
  Transmission/1(ImpellerTorque_[Nm]) -> Engine/1(ImpellerTorque_[Nm])  "ImpellerTorque_[Nm]"
  Gain/1 -> Bus Creator/1  "Vx_[kmh-1]"
  [RPM] -> Bus Creator/2  "NEngine_[rpm]"
  [gear] -> Bus Creator/3  "Gear_[-]"
  [ay] -> Bus Creator/5  "Ay_[ms-2]"
  [auto_manual] -> Bus Creator/6  "Auto_Manual_[-]"
  [throttle] -> Bus Creator/7  "Throttle_[perc]"
  [brake] -> Bus Creator/8  "Brake_[bar]"
  Engine/2(PEngine_[kW]) -> [PE]
  Bus Creator/1 -> Perf_Params/1
  [PE] -> Bus Creator/9  "PEngine_[kW]"
  Radians to Degrees/1 -> Bus Creator/11  "Roll_[deg]"
  Radians to Degrees1/1 -> Bus Creator/12  "Pitch_[deg]"
  [PD] -> Bus Creator/10  "PDrive_[kW]"
  Selector/1 -> Radians to Degrees/1
  Selector1/1 -> Radians to Degrees1/1
  [vx] -> Gain/1
  [ax] -> Bus Creator/4  "Ax_[ms-2]"

== system test_cs/Audi_A8_1/LKAS Controller ==
  note: State Feedback
  y : Inport
  -K : Gain  Gain=-K  Multiplication=Matrix(K*u)
  Mux1 : Mux
  Scope1 : Scope
  Scope2 : Scope  NumInputPorts=2
  State Feedback + Observer : Subsystem
  Sum1 : Sum  Inputs=|+-
  Steer [deg] : Outport
  wires:
  State Feedback + Observer/2(x2_hat) -> Mux1/2
  Sum1/1 -> State Feedback + Observer/2(y_hat)
  State Feedback + Observer/1(x1_hat) -> Mux1/1
  State Feedback + Observer/3(x3_hat) -> Mux1/3
  Mux1/1 -> -K/1  "X_hat"
  y/1 -> Sum1/1, Scope2/1
  State Feedback + Observer/4(x4_hat) -> Mux1/4, Scope2/2, Sum1/2  "y_hat"
  -K/1 -> State Feedback + Observer/1(Steer), Scope1/1, Steer [deg]/1

== system test_cs/Audi_A8_1/SELF_Demux ==
  SELF : Inport
  Demux1 : Demux  Outputs=3
  Demux2 : Demux  Outputs=3
  Demux3 : Demux  Outputs=[3 3 1 1]
  Demux4 : Demux  Outputs=3
  Gain : Gain  Gain=180/pi
  Gain1 : Gain  Gain=180/pi
  Selector : Selector  InputPortWidth=3  IndexOptions=Index vector (dialog)  Indices=[3]  OutputSizes=1
  compas converter : Subsystem
  xyz2GPS : S-Function  FunctionName=sfun_xyz2GPS  Parameters=CoordinateCount GPS_base  SFunctionDeploymentMode=off  EnableBusSupport=off  mask{CoordinateCount=1, GPS_base=[0.000000 0.000000 0.000]}
      mask prompts: CoordinateCount "Number of coordinates to convert"; GPS_base "GPS coordinate of the origin of the xyz coordinate system [lat lon alt]:"
      mask help:
      | Converts experiment xyz coordinates to GPS coordinates.
      |
      | The xyz coordinate system is defined as the tangential plane at the specified GPS coordinate (to be defined below), with x pointing east, y pointing north and z pointing to the outside of the earth.
      mask Display:
      | port_label('input', 1, 'x_{1},y_{1},z_{1},..,x_{N},y_{N},z_{N} [m]','texmode','on')
      | port_label('output', 1, 'Lat_{1},Lon_{1},Alt_{1},..,Lat_{N},Lon_{N},Alt_{N} [deg,deg,m]','texmode','on')
  x [m] : Outport
  y [m] : Outport  Port=2
  z [m] : Outport  Port=3
  rotx [deg] : Outport  Port=4
  roty [deg] : Outport  Port=5
  rotz [deg] : Outport  Port=6
  GPS lat [deg] : Outport  Port=7
  GPS long [deg] : Outport  Port=8
  GPS alt [m] : Outport  Port=9
  velocity [m/s] : Outport  Port=10
  heading [deg] : Outport  Port=11
  yaw rate [deg/s] : Outport  Port=12
  wires:
  Demux3/4 -> Gain1/1
  Gain1/1 -> yaw rate [deg/s]/1
  Demux3/3 -> velocity [m/s]/1
  compas converter/1(heading [deg]) -> heading [deg]/1
  xyz2GPS/1 -> Demux4/1
  Demux4/3 -> GPS alt [m]/1
  Demux4/2 -> GPS long [deg]/1
  Demux4/1 -> GPS lat [deg]/1
  Demux3/2 -> Gain/1, Selector/1
  Demux3/1 -> xyz2GPS/1, Demux1/1
  SELF/1 -> Demux3/1
  Demux2/3 -> rotz [deg]/1
  Demux2/2 -> roty [deg]/1
  Demux2/1 -> rotx [deg]/1
  Demux1/3 -> z [m]/1
  Demux1/2 -> y [m]/1
  Demux1/1 -> x [m]/1
  Gain/1 -> Demux2/1
  Selector/1 -> compas converter/1(rotz [rad])

== system test_cs/Audi_A8_1/Trajectories ==
  Traj2State1 : Subsystem  Tag=Traj2State  mask(PreScan Demux Block:){}
      settings: DeleteFcn=PreScanBlockDeleteFcn;
  Trajectory_1 : Subsystem  Tag=Trajectory  mask(PreScan Source Block: Trajectory){FileName='Trajectory_1.mat', TimeStep=1/20}
      mask prompts: TimeStep "Time Step [s]"
      mask help:
      | The Trajectory block contains the trajectories defined in the PreScan Experiment Editor. The output of the trajectory block is the (vehicle) State.
      |
      | For more information, please click Help.
      mask init:
      | [direc,name]=fileparts(get_param(bdroot, 'FileName'));
      | load([direc,'/Trajectories/',FileName])
      | trajectory=trajectory';
      | 
      | traj.time=trajectory(:,1);%[];
      | traj.signals.values=trajectory(:,2:19);
      | traj.dimensions=18;
      | traj.label='';
      | 
      | SampleTime=traj.time(2)-traj.time(1);
      settings: DeleteFcn=PreScanBlockDeleteFcn;
      mask Help: eval('openHelp(312)')
      mask Display: fprintf(FileName)
  Trajectory_1_Offset : Constant  Tag=TrajectoryOffset  Value="[0  0  0  0  0  0]"
  State : Outport  Tag=TrajOutport
  wires:
  Trajectory_1/1(trajectory) -> Traj2State1/1(Traj Org)  "L3"
  Trajectory_1_Offset/1 -> Traj2State1/2(Offset)  "L4"
  Traj2State1/1(state) -> State/1  "L5"

== system test_cs/STATE_Audi_A8_1/Acceleration ==
  Y : Inport
  Assignment : Assignment  IndexMode=Zero-based  SampleTime=TimeStep  IndexOptions=Starting index (dialog)  Indices=PortIndex  OutputSizes=[1 1]
  Data Store Read : DataStoreRead  DataStoreName=SimCoreActuators  SampleTime=TimeStep
  Data Store Write : DataStoreWrite  DataStoreName=SimCoreActuators
  wires:
  Assignment/1 -> Data Store Write/1
  Data Store Read/1 -> Assignment/1
  Y/1 -> Assignment/2

== system test_cs/STATE_Audi_A8_1/Position ==
  Y : Inport
  Assignment : Assignment  IndexMode=Zero-based  SampleTime=TimeStep  IndexOptions=Starting index (dialog)  Indices=PortIndex  OutputSizes=[1 1]
  Data Store Read : DataStoreRead  DataStoreName=SimCoreActuators  SampleTime=TimeStep
  Data Store Write : DataStoreWrite  DataStoreName=SimCoreActuators
  wires:
  Y/1 -> Assignment/2
  Data Store Read/1 -> Assignment/1
  Assignment/1 -> Data Store Write/1

== system test_cs/STATE_Audi_A8_1/RPY ==
  Y : Inport
  Assignment : Assignment  IndexMode=Zero-based  SampleTime=TimeStep  IndexOptions=Starting index (dialog)  Indices=PortIndex  OutputSizes=[1 1]
  Data Store Read : DataStoreRead  DataStoreName=SimCoreActuators  SampleTime=TimeStep
  Data Store Write : DataStoreWrite  DataStoreName=SimCoreActuators
  wires:
  Assignment/1 -> Data Store Write/1
  Data Store Read/1 -> Assignment/1
  Y/1 -> Assignment/2

== system test_cs/STATE_Audi_A8_1/Velocity ==
  Y : Inport
  Assignment : Assignment  IndexMode=Zero-based  SampleTime=TimeStep  IndexOptions=Starting index (dialog)  Indices=PortIndex  OutputSizes=[1 1]
  Data Store Read : DataStoreRead  DataStoreName=SimCoreActuators  SampleTime=TimeStep
  Data Store Write : DataStoreWrite  DataStoreName=SimCoreActuators
  wires:
  Assignment/1 -> Data Store Write/1
  Data Store Read/1 -> Assignment/1
  Y/1 -> Assignment/2

== system test_cs/STATE_Audi_A8_1/velRPY ==
  Y : Inport
  Assignment : Assignment  IndexMode=Zero-based  SampleTime=TimeStep  IndexOptions=Starting index (dialog)  Indices=PortIndex  OutputSizes=[1 1]
  Data Store Read : DataStoreRead  DataStoreName=SimCoreActuators  SampleTime=TimeStep
  Data Store Write : DataStoreWrite  DataStoreName=SimCoreActuators
  wires:
  Assignment/1 -> Data Store Write/1
  Data Store Read/1 -> Assignment/1
  Y/1 -> Assignment/2

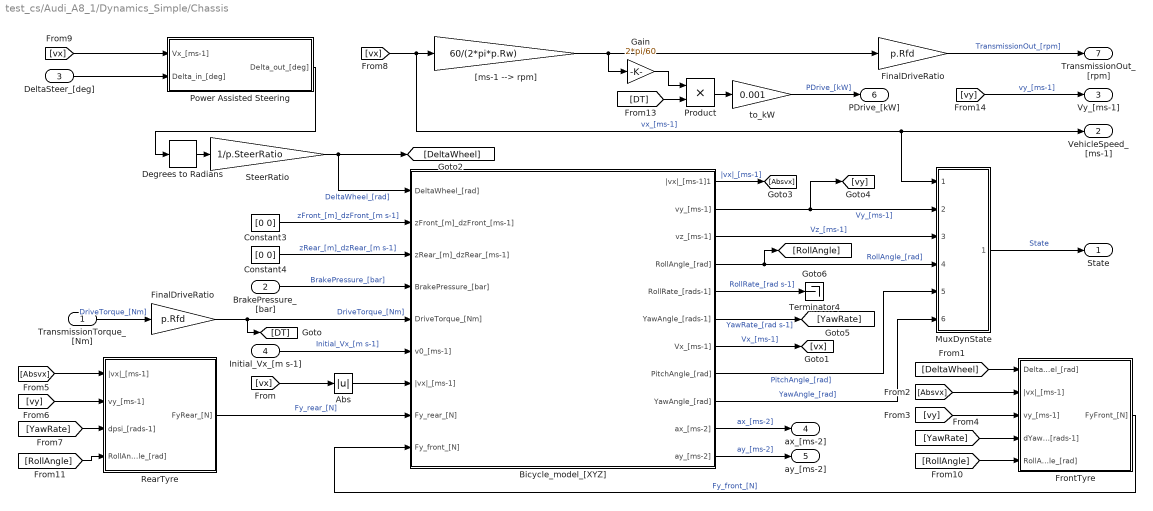
== system test_cs/Audi_A8_1/Dynamics_Simple/Chassis ==
  TransmissionTorque_[Nm] : Inport
  BrakePressure_[bar] : Inport  Port=2
  DeltaSteer_[deg] : Inport  Port=3
  Initial_Vx_[m s-1] : Inport  Port=4
  Abs : Abs
  Bicycle_model_[XYZ] : Subsystem
      mask Display: image(imread('Bicycle_model.png'));
  Constant3 : Constant  Value=[0 0]
  Constant4 : Constant  Value=[0 0]
  Degrees to Radians : simulink_extras/Transformations/Degrees to Radians
  FinalDriveRatio : Gain  Gain=p.Rfd  SaturateOnIntegerOverflow=on  OutDataTypeStr=Inherit: Same as input  ParamDataTypeStr=Inherit: Same as input
  "FinalDriveRatio " : Gain  Gain=p.Rfd  SaturateOnIntegerOverflow=on  OutDataTypeStr=Inherit: Same as input  ParamDataTypeStr=Inherit: Same as input
  FrontTyre : Subsystem
      mask Display: image(imread('Tyre.png'));
  Gain : Gain  Gain=2*pi/60
  MuxDynState : Subsystem
  Power Assisted Steering : Subsystem
  Product : Product  RndMeth=Zero
  RearTyre : Subsystem
      mask Display: image(imread('Tyre.png'));
  SteerRatio : Gain  Gain=1/p.SteerRatio
  Terminator4 : Terminator
  "[ms-1 --> rpm]" : Gain  Gain=60/(2*pi*p.Rw)  SaturateOnIntegerOverflow=on  OutDataTypeStr=Inherit: Same as input  ParamDataTypeStr=Inherit: Same as input
  to_kW : Gain  Gain=0.001
  State : Outport
  VehicleSpeed_[ms-1] : Outport  Port=2
  Vy_[ms-1] : Outport  Port=3
  ax_[ms-2] : Outport  Port=4
  ay_[ms-2] : Outport  Port=5
  PDrive_[kW] : Outport  Port=6
  TransmissionOut_[rpm] : Outport  Port=7
  wires:
  [vy] -> Vy_[ms-1]/1  "vy_[ms-1]"
  to_kW/1 -> PDrive_[kW]/1  "PDrive_[kW]"
  Gain/1 -> Product/1
  Bicycle_model_[XYZ]/10(ax_[ms-2]) -> ax_[ms-2]/1  "ax_[ms-2]"
  Product/1 -> to_kW/1
  [DT] -> Product/2
  Bicycle_model_[XYZ]/11(ay_[ms-2]) -> ay_[ms-2]/1  "ay_[ms-2]"
  Abs/1 -> Bicycle_model_[XYZ]/7(|vx|_[ms-1])
  Degrees to Radians/1 -> SteerRatio/1
  [vx] -> Abs/1
  SteerRatio/1 -> [DeltaWheel], Bicycle_model_[XYZ]/1(DeltaWheel_[rad])  "DeltaWheel_[rad]"
  TransmissionTorque_[Nm]/1 -> "FinalDriveRatio "/1  "DriveTorque_[Nm]"
  RearTyre/1(FyRear_[N]) -> Bicycle_model_[XYZ]/8(Fy_rear_[N])  "Fy_rear_[N]"
  FrontTyre/1(FyFront_[N]) -> Bicycle_model_[XYZ]/9(Fy_front_[N])  "Fy_front_[N]"
  Bicycle_model_[XYZ]/1(|vx|_[ms-1]1) -> [Absvx]  "|vx|_[ms-1]"
  Bicycle_model_[XYZ]/2(vy_[ms-1]) -> [vy], MuxDynState/2(vy [ms-1])  "Vy_[ms-1]"
  Bicycle_model_[XYZ]/4(RollAngle_[rad]) -> MuxDynState/4(R [rad]), [RollAngle]  "RollAngle_[rad]"
  Bicycle_model_[XYZ]/6(YawAngle_[rads-1]) -> [YawRate]  "YawRate_[rad s-1]"
  Bicycle_model_[XYZ]/7(Vx_[ms-1]) -> [vx]  "Vx_[ms-1]"
  [DeltaWheel] -> FrontTyre/1(DeltaWheel_[rad])
  [Absvx] -> FrontTyre/2(|vx|_[ms-1])
  [vy] -> FrontTyre/3(vy_[ms-1])
  [YawRate] -> FrontTyre/4(dYawAngle_[rads-1])
  [Absvx] -> RearTyre/1(|vx|_[ms-1])
  [vy] -> RearTyre/2(vy_[ms-1])
  [YawRate] -> RearTyre/3(dpsi_[rads-1])
  Bicycle_model_[XYZ]/3(vz_[ms-1]) -> MuxDynState/3(vz [ms-1])  "Vz_[ms-1]"
  Bicycle_model_[XYZ]/8(PitchAngle_[rad]) -> MuxDynState/5(P [rad])  "PitchAngle_[rad]"
  Bicycle_model_[XYZ]/9(YawAngle_[rad]) -> MuxDynState/6(Y [rad])  "YawAngle_[rad]"
  "[ms-1 --> rpm]"/1 -> Gain/1, FinalDriveRatio/1
  FinalDriveRatio/1 -> TransmissionOut_[rpm]/1  "TransmissionOut_[rpm]"
  [vx] -> "[ms-1 --> rpm]"/1, VehicleSpeed_[ms-1]/1, MuxDynState/1(vx [ms-1])  "vx_[ms-1]"
  [vx] -> Power Assisted Steering/1(Vx_[ms-1])
  DeltaSteer_[deg]/1 -> Power Assisted Steering/2(Delta_in_[deg])
  Power Assisted Steering/1(Delta_out_[deg]) -> Degrees to Radians/1
  [RollAngle] -> FrontTyre/5(RollAngle_[rad])
  [RollAngle] -> RearTyre/4(RollAngle_[rad])
  Constant3/1 -> Bicycle_model_[XYZ]/2(zFront_[m]_dzFront_[ms-1])  "zFront_[m]_dzFront_[m s-1]"
  Constant4/1 -> Bicycle_model_[XYZ]/3(zRear_[m]_dzRear_[ms-1])  "zRear_[m]_dzRear_[m s-1]"
  BrakePressure_[bar]/1 -> Bicycle_model_[XYZ]/4(BrakePressure_[bar])  "BrakePressure_[bar]"
  "FinalDriveRatio "/1 -> Bicycle_model_[XYZ]/5(DriveTorque_[Nm]), [DT]  "DriveTorque_[Nm]"
  Initial_Vx_[m s-1]/1 -> Bicycle_model_[XYZ]/6(v0_[ms-1])  "Initial_Vx_[m s-1]"
  Bicycle_model_[XYZ]/5(RollRate_[rads-1]) -> Terminator4/1  "RollRate_[rad s-1]"
  MuxDynState/1(State) -> State/1  "State"

== system test_cs/Audi_A8_1/Dynamics_Simple/Engine ==
  ImpellerTorque_[Nm] : Inport
  Throttle_[%] : Inport  Port=2
  Configurable Subsystem : Subsystem  BlockChoice=Rate Limiter  mask{ComputationMode=ComputationMode}
      mask prompts: ComputationMode "Compuation mode:"
      mask init:
      | SetComputationMode(gcb,ComputationMode);
      settings: AttributesFormatString=%<BlockChoice>  OpenFcn=BringToFront(gcb);  MemberBlocks=Discrete Rate Limiter,Rate Limiter
      settings: TemplateBlock=|
      | PreScanSimulinkLibrary/Configurable Subsystems/TransferFunction
      | Engine/Configurable
      | Subsystem
  Configurable Subsystem1 : Subsystem  BlockChoice=Integrator  mask{ComputationMode=ComputationMode}
      mask prompts: ComputationMode "Computation mode:"
      mask init:
      | SetComputationMode(gcb,ComputationMode);
      settings: AttributesFormatString=%<BlockChoice>  OpenFcn=BringToFront(gcb);  MemberBlocks=Discrete-Time Integrator,Integrator
      settings: TemplateBlock=|
      | PreScanSimulinkLibrary/Configurable Subsystems/integral with initial condition and limts
      | for engine/Configurable
      | Subsystem
  EngineTorque : Lookup2D  RowIndex=p.thvec  ColumnIndex=p.nevec  Table=p.emap  InputSameDT=on
  Gain : Gain  Gain=2*pi/60
  Product : Product  RndMeth=Zero
  Sum : Sum  Inputs=-+  SaturateOnIntegerOverflow=on  InputSameDT=on  OutDataTypeStr=Inherit: Same as first input
  engine + impeller inertia : Gain  Gain=1/p.Iei  SaturateOnIntegerOverflow=on  OutDataTypeStr=Inherit: Same as input  ParamDataTypeStr=Inherit: Same as input
  to_kW : Gain  Gain=0.001
  nEngine_[rpm] : Outport  InitialOutput=0
  PEngine_[kW] : Outport  Port=2  InitialOutput=0
  wires:
  EngineTorque/1 -> Sum/2, Product/2
  engine + impeller inertia/1 -> Configurable Subsystem1/1(In1)
  Sum/1 -> engine + impeller inertia/1
  Configurable Subsystem1/1(Out1) -> nEngine_[rpm]/1, EngineTorque/2, Gain/1  "rpm"
  Throttle_[%]/1 -> Configurable Subsystem/1(In1)
  ImpellerTorque_[Nm]/1 -> Sum/1
  Configurable Subsystem/1(Out1) -> EngineTorque/1
  Product/1 -> to_kW/1
  Gain/1 -> Product/1
  to_kW/1 -> PEngine_[kW]/1

== system test_cs/Audi_A8_1/Dynamics_Simple/Gear: Auto Manual ==
  note: 0; Auto = on // Manual =off
      | 1; Auto = off // Manual =on
  Auto_Manual : Inport
  Manual_Gear : Inport  Port=2
  Auto_Gear : Inport  Port=3
  If : If  IfExpression=u1 == 0
  If Action Subsystem : Subsystem  TreatAsAtomicUnit=on
  If Action Subsystem1 : Subsystem  TreatAsAtomicUnit=on
  Merge : Merge
  Gear : Outport
  wires:
  If Action Subsystem/1(Out1) -> Merge/1
  Auto_Gear/1 -> If Action Subsystem/1(In1)
  If/1 -> If Action Subsystem/Action
  Merge/1 -> Gear/1
  If Action Subsystem1/1(Out1) -> Merge/2
  Manual_Gear/1 -> If Action Subsystem1/1(In1)
  If/2 -> If Action Subsystem1/Action
  Auto_Manual/1 -> If/1

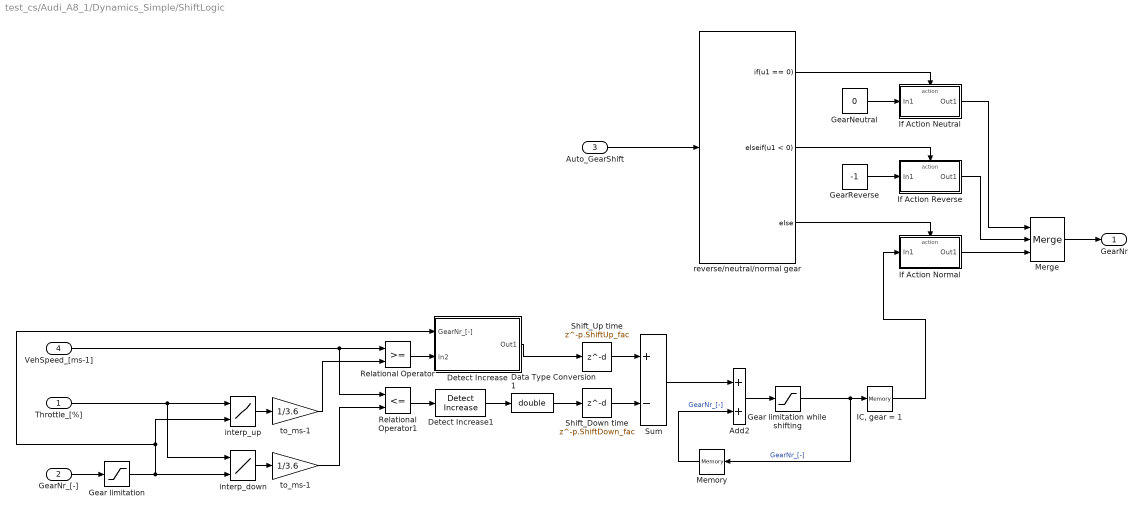
== system test_cs/Audi_A8_1/Dynamics_Simple/ShiftLogic ==
  Throttle_[%] : Inport
  GearNr_[-] : Inport  Port=2
  Auto_GearShift : Inport  Port=3
  VehSpeed_[ms-1] : Inport  Port=4
  Add2 : Sum
  Data Type Conversion1 : DataTypeConversion  OutDataTypeStr=double
  Detect Increase1 : simulink/Logic and Bit Operations/Detect Increase  vinit=0.0  InputProcessing=Inherited  OutDataTypeStr=uint8
  Detect Increase : Subsystem
  Gear limitation : Saturate  UpperLimit=p.maxGear  LowerLimit=1
  Gear limitation while shifting : Saturate  UpperLimit=p.maxGear  LowerLimit=1
  GearNeutral : Constant  Value=0
  GearReverse : Constant  Value=-1
  "IC, gear = 1" : Memory  X0=1  InheritSampleTime=on
  If Action Neutral : Subsystem  TreatAsAtomicUnit=on
  If Action Normal : Subsystem  TreatAsAtomicUnit=on
  If Action Reverse : Subsystem  TreatAsAtomicUnit=on
  Memory : Memory  InheritSampleTime=on
  Merge : Merge  Inputs=3
  Relational Operator : RelationalOperator  OutDataTypeStr=boolean  RndMeth=Nearest
  Relational Operator1 : RelationalOperator  Operator=<=  OutDataTypeStr=boolean  RndMeth=Nearest
  Shift_Down time : Delay  DelayLength=p.ShiftDown_fac  InputProcessing=Inherited
  Shift_Up time : Delay  DelayLength=p.ShiftUp_fac  InputProcessing=Inherited
  Sum : Sum  Inputs=+-
  interp_down : Lookup2D  RowIndex=p.downth  ColumnIndex=[1:p.maxGear]  Table=p.downtab  LookUpMeth=Interpolation-Use End Values  InputSameDT=on
  interp_up : Lookup2D  RowIndex=p.upth  ColumnIndex=[1:p.maxGear]  Table=p.uptab  LookUpMeth=Interpolation-Use End Values  InputSameDT=on
  reverse/neutral/normal gear : If  IfExpression=u1 == 0  ElseIfExpressions=u1 < 0
  to_ms-1 : Gain  Gain=1/3.6
  "to_ms-1 " : Gain  Gain=1/3.6
  GearNr : Outport
  wires:
  Auto_GearShift/1 -> reverse/neutral/normal gear/1
  "IC, gear = 1"/1 -> If Action Normal/1(In1)
  Merge/1 -> GearNr/1
  If Action Reverse/1(Out1) -> Merge/2
  If Action Neutral/1(Out1) -> Merge/1
  If Action Normal/1(Out1) -> Merge/3
  reverse/neutral/normal gear/3 -> If Action Normal/Action
  reverse/neutral/normal gear/1 -> If Action Neutral/Action
  reverse/neutral/normal gear/2 -> If Action Reverse/Action
  GearReverse/1 -> If Action Reverse/1(In1)
  GearNeutral/1 -> If Action Neutral/1(In1)
  Shift_Down time/1 -> Sum/2
  Shift_Up time/1 -> Sum/1
  Detect Increase/1(Out1) -> Shift_Up time/1
  Data Type Conversion1/1 -> Shift_Down time/1
  Detect Increase1/1 -> Data Type Conversion1/1
  Sum/1 -> Add2/1
  Memory/1 -> Add2/2  "GearNr_[-]"
  Add2/1 -> Gear limitation while shifting/1
  Gear limitation while shifting/1 -> "IC, gear = 1"/1, Memory/1  "GearNr_[-]"
  Throttle_[%]/1 -> interp_down/1, interp_up/1
  Relational Operator/1 -> Detect Increase/2(In2)
  Relational Operator1/1 -> Detect Increase1/1
  interp_down/1 -> "to_ms-1 "/1
  VehSpeed_[ms-1]/1 -> Relational Operator/1, Relational Operator1/1
  interp_up/1 -> to_ms-1/1
  Gear limitation/1 -> interp_down/2, interp_up/2, Detect Increase/1(GearNr_[-])
  GearNr_[-]/1 -> Gear limitation/1
  to_ms-1/1 -> Relational Operator/2
  "to_ms-1 "/1 -> Relational Operator1/2

== system test_cs/Audi_A8_1/Dynamics_Simple/Transmission ==
  nEngine_[rpm] : Inport
  GearNr_[-] : Inport  Port=2
  n_TransmissionOut_[rpm] : Inport  Port=3
  Torque_Converter : Subsystem
      mask Display: image(imread('TorqueConverter.png'));
  Transmission_Ratio : Subsystem
  Viscous coupling : Lookup  InputValues=[-5:0.1:5]*p.m/4  Table=p.m/4*tanh([-5:0.1:5])
  ImpellerTorque_[Nm] : Outport  InitialOutput=0
  TransmissionTorque_[Nm] : Outport  Port=2  InitialOutput=0
  wires:
  Torque_Converter/2(TurbineTorque_[Nm]) -> Viscous coupling/1  "Converter_Torque_[Nm]"
  Transmission_Ratio/2(nTransmissionIn_[rpm]) -> Torque_Converter/2(nTransmission_[rpm])
  nEngine_[rpm]/1 -> Torque_Converter/1(nEngine_[rpm])
  GearNr_[-]/1 -> Transmission_Ratio/2(GearNr_[-]), Torque_Converter/3(Gear nr)
  n_TransmissionOut_[rpm]/1 -> Transmission_Ratio/3(nTransmissionOut_[rpm])
  Torque_Converter/1(ImpellerTorque_[Nm]) -> ImpellerTorque_[Nm]/1
  Transmission_Ratio/1(tTransmissionOut_[Nm]) -> TransmissionTorque_[Nm]/1
  Viscous coupling/1 -> Transmission_Ratio/1(tTransmissionIn_[Nm])

== system test_cs/Audi_A8_1/LKAS Controller/State Feedback + Observer ==
  note: lateral_offset
  note: lateral_offset_dot
  note: yaw
  note: yaw_rate
  Steer : Inport
  y_hat : Inport  Port=2
  Differential Equation : Subsystem
  x1_hat : Outport
  x2_hat : Outport  Port=2
  x3_hat : Outport  Port=3
  x4_hat : Outport  Port=4
  wires:
  Differential Equation/1(x1_hat) -> x1_hat/1
  Differential Equation/4(x4_hat) -> x4_hat/1
  y_hat/1 -> Differential Equation/2(y_hat)
  Steer/1 -> Differential Equation/1(Steer)
  Differential Equation/2(x2_hat) -> x2_hat/1
  Differential Equation/3(x3_hat) -> x3_hat/1

== system test_cs/Audi_A8_1/SELF_Demux/compas converter ==
  rotz [rad] : Inport
  cart2compas : Subsystem
  rad2deg : Gain  Gain=180/pi
  heading [deg] : Outport
  wires:
  cart2compas/1(heading [deg]) -> heading [deg]/1
  rotz [rad]/1 -> rad2deg/1
  rad2deg/1 -> cart2compas/1(Angle [deg])

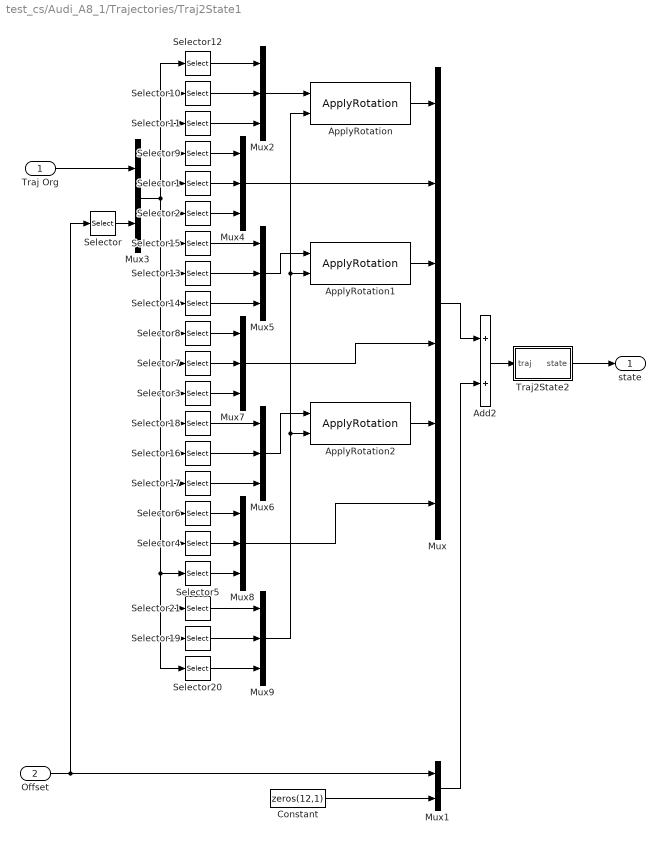
== system test_cs/Audi_A8_1/Trajectories/Traj2State1 ==
  Traj Org : Inport
  Offset : Inport  Port=2
  Add2 : Sum
  ApplyRotation : PreScanSimulinkLibrary/ApplyRotation
  ApplyRotation1 : PreScanSimulinkLibrary/ApplyRotation
  ApplyRotation2 : PreScanSimulinkLibrary/ApplyRotation
  Constant : Constant  Value=zeros(12,1)
  Mux : Mux  Inputs=6
  Mux1 : Mux  Inputs=2
  Mux{2,4..9} (7 alike) : Mux  Inputs=3
  Mux3 : Mux  Inputs=2
  Selector : Selector  InputPortWidth=6  IndexOptions=Index vector (dialog)  Indices=[4 5 6]  OutputSizes=1
  Selector1 : Selector  InputPortWidth=21  IndexOptions=Index vector (dialog)  Indices=[5]  OutputSizes=1
  Selector10 : Selector  InputPortWidth=21  IndexOptions=Index vector (dialog)  Indices=[2]  OutputSizes=1
  Selector11 : Selector  InputPortWidth=21  IndexOptions=Index vector (dialog)  Indices=[3]  OutputSizes=1
  Selector12 : Selector  InputPortWidth=21  IndexOptions=Index vector (dialog)  Indices=[1]  OutputSizes=1
  Selector13 : Selector  InputPortWidth=21  IndexOptions=Index vector (dialog)  Indices=[8]  OutputSizes=1
  Selector14 : Selector  InputPortWidth=21  IndexOptions=Index vector (dialog)  Indices=[9]  OutputSizes=1
  Selector15 : Selector  InputPortWidth=21  IndexOptions=Index vector (dialog)  Indices=[7]  OutputSizes=1
  Selector16 : Selector  InputPortWidth=21  IndexOptions=Index vector (dialog)  Indices=[14]  OutputSizes=1
  Selector17 : Selector  InputPortWidth=21  IndexOptions=Index vector (dialog)  Indices=[15]  OutputSizes=1
  Selector18 : Selector  InputPortWidth=21  IndexOptions=Index vector (dialog)  Indices=[13]  OutputSizes=1
  Selector19 : Selector  InputPortWidth=21  IndexOptions=Index vector (dialog)  Indices=[20]  OutputSizes=1
  Selector2 : Selector  InputPortWidth=21  IndexOptions=Index vector (dialog)  Indices=[6]  OutputSizes=1
  Selector20 : Selector  InputPortWidth=21  IndexOptions=Index vector (dialog)  Indices=[21]  OutputSizes=1
  Selector21 : Selector  InputPortWidth=21  IndexOptions=Index vector (dialog)  Indices=[19]  OutputSizes=1
  Selector3 : Selector  InputPortWidth=21  IndexOptions=Index vector (dialog)  Indices=[12]  OutputSizes=1
  Selector4 : Selector  InputPortWidth=21  IndexOptions=Index vector (dialog)  Indices=[17]  OutputSizes=1
  Selector5 : Selector  InputPortWidth=21  IndexOptions=Index vector (dialog)  Indices=[18]  OutputSizes=1
  Selector6 : Selector  InputPortWidth=21  IndexOptions=Index vector (dialog)  Indices=[16]  OutputSizes=1
  Selector7 : Selector  InputPortWidth=21  IndexOptions=Index vector (dialog)  Indices=[11]  OutputSizes=1
  Selector8 : Selector  InputPortWidth=21  IndexOptions=Index vector (dialog)  Indices=[10]  OutputSizes=1
  Selector9 : Selector  InputPortWidth=21  IndexOptions=Index vector (dialog)  Indices=[4]  OutputSizes=1
  Traj2State2 : Subsystem
  state : Outport
  wires:
  Mux9/1 -> ApplyRotation2/2, ApplyRotation1/2, ApplyRotation/2
  Selector20/1 -> Mux9/3
  Selector19/1 -> Mux9/2
  Selector21/1 -> Mux9/1
  Selector5/1 -> Mux8/3
  Selector4/1 -> Mux8/2
  Selector6/1 -> Mux8/1
  Mux8/1 -> Mux/6
  Mux6/1 -> ApplyRotation2/1
  Mux7/1 -> Mux/4
  ApplyRotation2/1 -> Mux/5
  Selector3/1 -> Mux7/3
  Selector7/1 -> Mux7/2
  Selector8/1 -> Mux7/1
  Mux4/1 -> Mux/2
  Mux5/1 -> ApplyRotation1/1
  ApplyRotation1/1 -> Mux/3
  Mux2/1 -> ApplyRotation/1
  ApplyRotation/1 -> Mux/1
  Selector2/1 -> Mux4/3
  Selector1/1 -> Mux4/2
  Selector9/1 -> Mux4/1
  Selector17/1 -> Mux6/3
  Selector16/1 -> Mux6/2
  Selector18/1 -> Mux6/1
  Selector14/1 -> Mux5/3
  Selector13/1 -> Mux5/2
  Selector15/1 -> Mux5/1
  Selector11/1 -> Mux2/3
  Selector10/1 -> Mux2/2
  Selector12/1 -> Mux2/1
  Mux3/1 -> Selector8/1, Selector7/1, Selector3/1, Selector18/1, Selector16/1, Selector17/1, Selector6/1, Selector20/1, Selector19/1, Selector21/1, Selector5/1, Selector4/1, Selector14/1, Selector13/1, Selector15/1, Selector2/1, Selector1/1, Selector9/1, Selector12/1, Selector10/1, Selector11/1
  Mux1/1 -> Add2/2
  Constant/1 -> Mux1/2
  Add2/1 -> Traj2State2/1(traj)
  Selector/1 -> Mux3/2
  Traj Org/1 -> Mux3/1
  Offset/1 -> Mux1/1, Selector/1
  Mux/1 -> Add2/1
  Traj2State2/1(state) -> state/1

== system test_cs/Audi_A8_1/Trajectories/Trajectory_1 ==
  From Workspace : FromWorkspace  VariableName=trajectory  SampleTime=TimeStep  OutputAfterFinalValue=Holding final value
  From Workspace1 : FromWorkspace  VariableName=trajectory  SampleTime=TimeStep  OutputAfterFinalValue=Setting to zero
  Mux : Mux  Inputs=2
  Selector1 : Selector  InputPortWidth=24  IndexOptions=Index vector (dialog)  Indices=[7:18]  OutputSizes=1
  Selector9 : Selector  InputPortWidth=24  IndexOptions=Index vector (dialog)  Indices=[1:6]  OutputSizes=1
  trajectory : Outport
  wires:
  Selector1/1 -> Mux/2
  Selector9/1 -> Mux/1
  Mux/1 -> trajectory/1
  From Workspace1/1 -> Selector1/1
  From Workspace/1 -> Selector9/1
